simulink model "torqueControlBalancingWithSimu"  (Simulink 10.2)
settings: Solver=FixedStepDiscrete  StartTime=0.0  StopTime="Config.SIMULATION_TIME "  FixedStep=Config.tStepSim  RelTol=1e-3
PostLoadFcn:
  | %% Try to open the static GUI and try to adjust it
  | try
  | 
  |     staticGUI = simulinkStaticGUI;
  | 
  | end
InitFcn:
  | %% initialize the simulation
  | cd(fileparts(which(bdroot)));
  | initTorqueControlBalancingWithSimu;
  | 
  | %% Try to edit the GUI (the user may have already closed it)
  | try
  | 
  |     %% Update Start Button
  |     set(sl_synch_handles.startButton,'Backgroundcolor',[0.0,1.0,0.0]);
  |     set(sl_synch_handles.startButton,'Enable','on');
  | 
  | end
StartFcn:
  | %% Try to edit the GUI (the user may have already closed it)
  | try
  | 
  |     %% Update Start Button
  |     set(sl_synch_handles.startButton,'Backgroundcolor',[0.8,0.8,0.8]);
  |     set(sl_synch_handles.startButton,'Enable','off');
  | 
  |     %% Update Compile Button
  |     set(sl_synch_handles.compileButton,'Backgroundcolor',[0.8,0.8,0.8]);
  |     set(sl_synch_handles.compileButton,'Enable','off');
  | 
  |     %% Update Exit Button
  |     set(sl_synch_handles.exitButton,'Backgroundcolor',[0.8,0.8,0.8]);
  |     set(sl_synch_handles.exitButton,'Enable','off');
  | 
  | end
StopFcn:
  | %% stop the simulation
  | cd(fileparts(which(bdroot)));
  | stopTorqueControlBalancingWithSimu;
  | 
  | %% Try to edit the GUI (the user may have already closed it)
  | try
  | 
  |     %% Update Start Button
  |     if get(sl_synch_handles.checkbox_recompile, 'Value')
  |         set(sl_synch_handles.startButton,'Backgroundcolor',[0.0,1.0,0.0]);
  |         set(sl_synch_handles.startButton,'Enable','on');
  |     end
  | 
  |     %% Update Compile Button
  |     set(sl_synch_handles.compileButton,'Backgroundcolor',[1.0,0.6,0.0]);
  |     set(sl_synch_handles.compileButton,'Enable','on');
  | 
  |     %% Update Exit Button
  |     set(sl_synch_handles.exitButton,'Backgroundcolor',[0.0,1.0,1.0]);
  |     set(sl_synch_handles.exitButton,'Enable','on');
  | 
  | end
undefined symbols (not defined in the file or in its folder): bVectorConstraints, Config, confVisualizer, ConstraintsMatrix, Gain, motorsReflectedInertia, Reg, robot_config, ROBOT_DOF, Sat, StateMachine
libraries: WBToolboxLibrary x36, utilityBlocks_lib x7, mwbs_visualizers_lib x1, mwbs_robotSensors_lib x1, mwbs_robotDynamicsWithContacts_lib x1
(part 2 of 2)

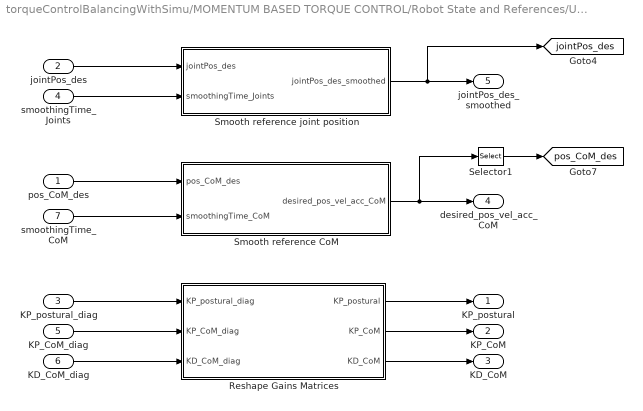
== system torqueControlBalancingWithSimu/MOMENTUM BASED TORQUE CONTROL/Robot State and References/Update Gains and References ==
  pos_CoM_des : Inport
  jointPos_des : Inport  Port=2
  KP_postural_diag : Inport  Port=3
  smoothingTime_Joints : Inport  Port=4
  KP_CoM_diag : Inport  Port=5
  KD_CoM_diag : Inport  Port=6
  smoothingTime_CoM : Inport  Port=7
  Reshape Gains Matrices : Subsystem
  Selector1 : Selector  NumberOfDimensions=2  InputPortWidth=3  IndexOptions=Index vector (dialog),Index vector (dialog)  Indices=[1 2 3],[1]  OutputSizes=1,1
  Smooth reference CoM : Subsystem
  Smooth reference joint position : Subsystem
  KP_postural : Outport  VectorParamsAs1DForOutWhenUnconnected=off
  KP_CoM : Outport  Port=2  VectorParamsAs1DForOutWhenUnconnected=off
  KD_CoM : Outport  Port=3  VectorParamsAs1DForOutWhenUnconnected=off
  desired_pos_vel_acc_CoM : Outport  Port=4  VectorParamsAs1DForOutWhenUnconnected=off
  jointPos_des_smoothed : Outport  Port=5  VectorParamsAs1DForOutWhenUnconnected=off
  tag scope: jointPos_des=global, pos_CoM_des=global
  wires:
  Smooth reference joint position/1(jointPos_des_smoothed) -> [jointPos_des], jointPos_des_smoothed/1
  jointPos_des/1 -> Smooth reference joint position/1(jointPos_des)
  smoothingTime_Joints/1 -> Smooth reference joint position/2(smoothingTime_Joints)
  pos_CoM_des/1 -> Smooth reference CoM/1(pos_CoM_des)
  smoothingTime_CoM/1 -> Smooth reference CoM/2(smoothingTime_CoM)
  Smooth reference CoM/1(desired_pos_vel_acc_CoM) -> Selector1/1, desired_pos_vel_acc_CoM/1
  KP_postural_diag/1 -> Reshape Gains Matrices/1(KP_postural_diag)
  KP_CoM_diag/1 -> Reshape Gains Matrices/2(KP_CoM_diag)
  KD_CoM_diag/1 -> Reshape Gains Matrices/3(KD_CoM_diag)
  Reshape Gains Matrices/1(KP_postural) -> KP_postural/1
  Reshape Gains Matrices/2(KP_CoM) -> KP_CoM/1
  Reshape Gains Matrices/3(KD_CoM) -> KD_CoM/1
  Selector1/1 -> [pos_CoM_des]

== system torqueControlBalancingWithSimu/MOMENTUM BASED TORQUE CONTROL/emergency stop: joint limits/STOP IF JOINTS HIT THE LIMITS ==
  jointPos : Inport
  Enable : EnablePort
  Assertion : Assertion
  GetLimits : WBToolboxLibrary/States/GetLimits  limitsSource=ControlBoard  limitsType=Position
      settings: SourceProductName=WholeBodyToolbox
  MATLAB Function : MATLAB Function  TreatAsAtomicUnit=on
  To Workspace : ToWorkspace  VariableName=res_check_range  SaveFormat=Structure With Time  SampleTime=Config.tStep
  Unit Delay : UnitDelay  InitialCondition=1  SampleTime=Config.tStep  HasFrameUpgradeWarning=on
  index1 : Constant  Value=0.01  VectorParams1D=off
  wires:
  jointPos/1 -> MATLAB Function/3(u)
  MATLAB Function/1(inRange) -> Unit Delay/1
  index1/1 -> MATLAB Function/4(tol)
  MATLAB Function/2(res_check_range) -> To Workspace/1
  Unit Delay/1 -> Assertion/1
  GetLimits/1 -> MATLAB Function/1(umin)
  GetLimits/2 -> MATLAB Function/2(umax)

== system torqueControlBalancingWithSimu/MOMENTUM BASED TORQUE CONTROL/emergency stop: joint limits/STOP IF THERE ARE SPIKES IN THE ENCODERS ==
  jointPos : Inport
  Enable : EnablePort
  Assertion : Assertion
  MATLAB Function : MATLAB Function  TreatAsAtomicUnit=on
  To Workspace : ToWorkspace  VariableName=res_check_spikes  SaveFormat=Structure With Time  SampleTime=Config.tStep
  Unit Delay : UnitDelay  InitialCondition=1  SampleTime=Config.tStep  HasFrameUpgradeWarning=on
  index1 : Constant  Value=Sat.maxJointsPositionDelta  VectorParams1D=off
  wires:
  jointPos/1 -> MATLAB Function/1(u)
  MATLAB Function/1(noSpikes) -> Unit Delay/1
  index1/1 -> MATLAB Function/2(delta_u_max)
  MATLAB Function/2(res_check_spikes) -> To Workspace/1
  Unit Delay/1 -> Assertion/1

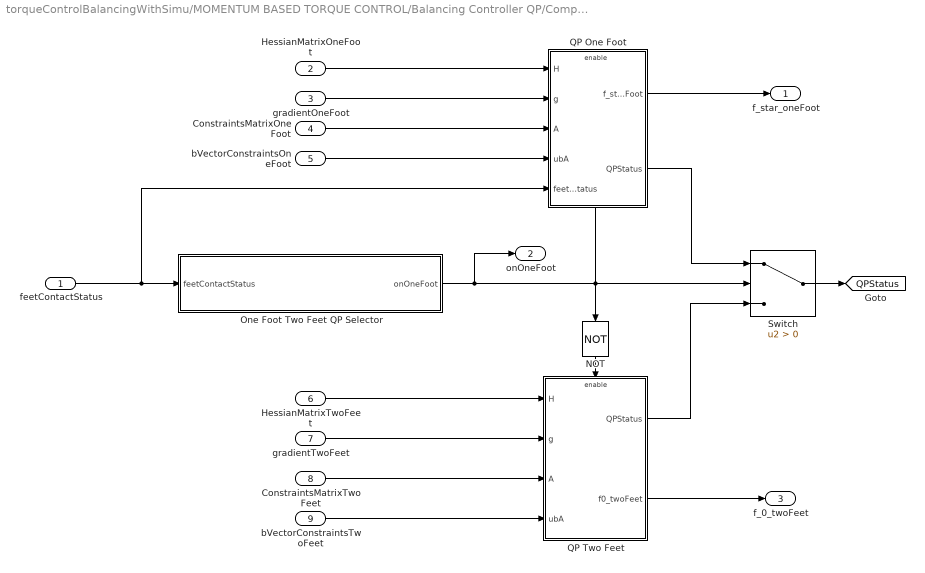
== system torqueControlBalancingWithSimu/MOMENTUM BASED TORQUE CONTROL/Balancing Controller QP/Compute Desired Torques/QPSolver ==
  feetContactStatus : Inport
  HessianMatrixOneFoot : Inport  Port=2
  gradientOneFoot : Inport  Port=3
  ConstraintsMatrixOneFoot : Inport  Port=4
  bVectorConstraintsOneFoot : Inport  Port=5
  HessianMatrixTwoFeet : Inport  Port=6
  gradientTwoFeet : Inport  Port=7
  ConstraintsMatrixTwoFeet : Inport  Port=8
  bVectorConstraintsTwoFeet : Inport  Port=9
  NOT : Logic  Operator=NOT  IconShape=distinctive  AllPortsSameDT=off  OutDataTypeStr=boolean
  One Foot Two Feet QP Selector : MATLAB Function  TreatAsAtomicUnit=on
  QP One Foot : Subsystem  TreatAsAtomicUnit=on
  QP Two Feet : Subsystem  TreatAsAtomicUnit=on
  Switch : Switch  Criteria=u2 > Threshold
  f_star_oneFoot : Outport  VectorParamsAs1DForOutWhenUnconnected=off
  onOneFoot : Outport  Port=2  VectorParamsAs1DForOutWhenUnconnected=off
  f_0_twoFeet : Outport  Port=3  VectorParamsAs1DForOutWhenUnconnected=off
  tag scope: QPStatus=global
  wires:
  feetContactStatus/1 -> QP One Foot/5(feetContactStatus), One Foot Two Feet QP Selector/1(feetContactStatus)
  HessianMatrixOneFoot/1 -> QP One Foot/1(H)
  bVectorConstraintsTwoFeet/1 -> QP Two Feet/4(ubA)
  gradientOneFoot/1 -> QP One Foot/2(g)
  ConstraintsMatrixOneFoot/1 -> QP One Foot/3(A)
  gradientTwoFeet/1 -> QP Two Feet/2(g)
  ConstraintsMatrixTwoFeet/1 -> QP Two Feet/3(A)
  bVectorConstraintsOneFoot/1 -> QP One Foot/4(ubA)
  HessianMatrixTwoFeet/1 -> QP Two Feet/1(H)
  QP One Foot/2(QPStatus) -> Switch/1
  QP Two Feet/1(QPStatus) -> Switch/3
  QP Two Feet/2(f0_twoFeet) -> f_0_twoFeet/1
  NOT/1 -> QP Two Feet/Enable
  One Foot Two Feet QP Selector/1(onOneFoot) -> onOneFoot/1, NOT/1, Switch/2, QP One Foot/Enable
  QP One Foot/1(f_star_oneFoot) -> f_star_oneFoot/1
  Switch/1 -> [QPStatus]

== system torqueControlBalancingWithSimu/MOMENTUM BASED TORQUE CONTROL/Balancing Controller QP/Compute angular momentum integral error/Compute base to fixed link transform ==
  jointPos : Inport
  Constant7 : Constant  Value=eye(4)
  "inv  " : Product  Inputs=/  Multiplication=Matrix(*)
  inv  1 : Product  Inputs=/  Multiplication=Matrix(*)
  l_sole to root_link relative transform : WBToolboxLibrary/Model/Kinematics/ForwardKinematics  frameName=Frames.LEFT_FOOT
      settings: SourceProductName=WholeBodyToolbox
  r_sole to root_link relative transform : WBToolboxLibrary/Model/Kinematics/ForwardKinematics  frameName=Frames.RIGHT_FOOT
      settings: SourceProductName=WholeBodyToolbox
  fixed_l_sole_H_b : Outport  VectorParamsAs1DForOutWhenUnconnected=off
  fixed_r_sole_H_b : Outport  Port=2  VectorParamsAs1DForOutWhenUnconnected=off
  wires:
  Constant7/1 -> l_sole to root_link relative transform/1, r_sole to root_link relative transform/1
  inv  1/1 -> fixed_r_sole_H_b/1
  "inv  "/1 -> fixed_l_sole_H_b/1
  jointPos/1 -> r_sole to root_link relative transform/2, l_sole to root_link relative transform/2
  l_sole to root_link relative transform/1 -> "inv  "/1
  r_sole to root_link relative transform/1 -> inv  1/1

== system torqueControlBalancingWithSimu/MOMENTUM BASED TORQUE CONTROL/Dump and visualize/Desired and Measured Forces/Demux Forces nd Moments ==
  wrench_leftFoot : Inport
  wrench_rightFoot : Inport  Port=2
  f_star : Inport  Port=3
  Demux{1,5..7} (4 alike) : Demux  Outputs=[3;3]
  Demux2 : Demux  Outputs=[6;6]
  measured forces l_sole : Outport  VectorParamsAs1DForOutWhenUnconnected=off
  des forces l_sole : Outport  Port=2  VectorParamsAs1DForOutWhenUnconnected=off
  measured forces r_sole : Outport  Port=3  VectorParamsAs1DForOutWhenUnconnected=off
  des forces r_sole : Outport  Port=4  VectorParamsAs1DForOutWhenUnconnected=off
  measured moments l_sole : Outport  Port=5  VectorParamsAs1DForOutWhenUnconnected=off
  des moments l_sole : Outport  Port=6  VectorParamsAs1DForOutWhenUnconnected=off
  measured moments r_sole : Outport  Port=7  VectorParamsAs1DForOutWhenUnconnected=off
  des moments r_sole : Outport  Port=8  VectorParamsAs1DForOutWhenUnconnected=off
  wires:
  Demux6/2 -> des moments r_sole/1
  Demux5/2 -> des moments l_sole/1
  Demux1/1 -> measured forces l_sole/1
  Demux7/1 -> measured forces r_sole/1
  Demux7/2 -> measured moments r_sole/1
  wrench_leftFoot/1 -> Demux1/1
  Demux2/1 -> Demux5/1
  wrench_rightFoot/1 -> Demux7/1
  Demux6/1 -> des forces r_sole/1
  Demux1/2 -> measured moments l_sole/1
  f_star/1 -> Demux2/1
  Demux2/2 -> Demux6/1
  Demux5/1 -> des forces l_sole/1

== system torqueControlBalancingWithSimu/MOMENTUM BASED TORQUE CONTROL/Dynamics and Kinematics/Dynamics/Add motors reflected inertia ==
  M : Inport
  Add motor reflected inertias : MATLAB Function  TreatAsAtomicUnit=on
  Constant : Constant  Value=Config.USE_MOTOR_REFLECTED_INERTIA
  Switch : Switch  Criteria=u2 > Threshold
  M_with_motor_inertia : Outport  VectorParamsAs1DForOutWhenUnconnected=off
  wires:
  M/1 -> Switch/3, Add motor reflected inertias/1(M)
  Constant/1 -> Switch/2
  Add motor reflected inertias/1(M_with_inertia) -> Switch/1
  Switch/1 -> M_with_motor_inertia/1

== system torqueControlBalancingWithSimu/MOMENTUM BASED TORQUE CONTROL/Robot State and References/Compute State Velocity/Feet Jacobians ==
  jointPos : Inport
  w_H_b : Inport  Port=2
  Jacobian l_sole : WBToolboxLibrary/Model/Jacobians/Jacobian  frameName=Frames.LEFT_FOOT
      settings: SourceProductName=WholeBodyToolbox
  Jacobian r_sole : WBToolboxLibrary/Model/Jacobians/Jacobian  frameName=Frames.RIGHT_FOOT
      settings: SourceProductName=WholeBodyToolbox
  J_l_sole : Outport  VectorParamsAs1DForOutWhenUnconnected=off
  J_r_sole : Outport  Port=2  VectorParamsAs1DForOutWhenUnconnected=off
  wires:
  Jacobian l_sole/1 -> J_l_sole/1
  Jacobian r_sole/1 -> J_r_sole/1
  w_H_b/1 -> Jacobian r_sole/1, Jacobian l_sole/1
  jointPos/1 -> Jacobian l_sole/2, Jacobian r_sole/2

== system torqueControlBalancingWithSimu/MOMENTUM BASED TORQUE CONTROL/Robot State and References/Compute base to fixed link transform/LFoot to base link transform  ==
  neck_pos : Inport
  jointPos : Inport  Port=2
  inertial : Inport  Port=3
  w_H_link : Inport  Port=4
  w_H_base_fixed : Inport  Port=5
  Fixe d base to root link transform : WBToolboxLibrary/Model/Kinematics/ForwardKinematics  frameName=Frames.BASE
      settings: SourceProductName=WholeBodyToolbox
  Fixed base to imu transform : WBToolboxLibrary/Model/Kinematics/ForwardKinematics  frameName=Frames.IMU
      settings: SourceProductName=WholeBodyToolbox
  Get Base Rotation From IMU : MATLAB Function  TreatAsAtomicUnit=on
  Inv : Product  Inputs=/*  Multiplication=Matrix(*)
  Inv_2 : Product  Inputs=/*  Multiplication=Matrix(*)
  Selector1 : Selector  InputPortWidth=Ports.IMU_PORT_SIZE  IndexOptions=Index vector (dialog)  Indices=Ports.IMU_PORT_ORIENTATION_INDEX  OutputSizes=1
  Selector2 : Selector  InputPortWidth=Ports.IMU_PORT_SIZE  IndexOptions=Index vector (dialog)  Indices=Ports.IMU_PORT_ORIENTATION_INDEX  OutputSizes=1
  Switch6 : Switch  Criteria=u2 > Threshold
  USE_IMU4EST_BASE : Constant  Value=Config.USE_IMU4EST_BASE
  holder 1 : utilityBlocks_lib/Holder  SystemSampleTime=Config.tStep  VariantActivationTime=update diagram  Latency=0  AutoFrameSizeCalculation=off
      settings: SourceProductName=WholeBodyControllers
  holder 2 : utilityBlocks_lib/Holder  SystemSampleTime=Config.tStep  VariantActivationTime=update diagram  Latency=0  AutoFrameSizeCalculation=off
      settings: SourceProductName=WholeBodyControllers
  neck transform : Subsystem
  link_H_b : Outport  VectorParamsAs1DForOutWhenUnconnected=off
  wires:
  Switch6/1 -> link_H_b/1
  Inv_2/1 -> Switch6/3, Get Base Rotation From IMU/3(fixedLink_H_base)  "link_H_root"
  USE_IMU4EST_BASE/1 -> Switch6/2
  Inv/1 -> holder 1/1, Get Base Rotation From IMU/1(imu_H_fixedLink)  "imu_H_link"
  holder 2/1 -> Selector2/1
  Fixed base to imu transform/1 -> Inv/1
  jointPos/1 -> Fixed base to imu transform/2, Fixe d base to root link transform/2
  Get Base Rotation From IMU/1(w_H_b) -> Switch6/1
  Fixe d base to root link transform/1 -> Inv_2/2
  inertial/1 -> Selector1/1, holder 2/1
  neck_pos/1 -> neck transform/1(neck port)
  w_H_link/1 -> Inv_2/1, Inv/2
  w_H_base_fixed/1 -> Fixe d base to root link transform/1, Fixed base to imu transform/1
  Selector2/1 -> Get Base Rotation From IMU/4(rpyFromIMU_0)
  holder 1/1 -> Get Base Rotation From IMU/2(imu_H_fixedLink_0)
  Selector1/1 -> Get Base Rotation From IMU/5(rpyFromIMU)
  neck transform/1(neck position) -> Get Base Rotation From IMU/6(neck_pos)

== system torqueControlBalancingWithSimu/MOMENTUM BASED TORQUE CONTROL/Robot State and References/Compute base to fixed link transform/RFoot to base link transform ==
  neck_pos : Inport
  jointPos : Inport  Port=2
  inertial : Inport  Port=3
  w_H_link : Inport  Port=4
  w_H_base_fixed : Inport  Port=5
  Fixed base to imu transform : WBToolboxLibrary/Model/Kinematics/ForwardKinematics  frameName=Frames.IMU
      settings: SourceProductName=WholeBodyToolbox
  Fixed base to root link transform : WBToolboxLibrary/Model/Kinematics/ForwardKinematics  frameName=Frames.BASE
      settings: SourceProductName=WholeBodyToolbox
  Get Base Rotation From IMU : MATLAB Function  TreatAsAtomicUnit=on
  Inv : Product  Inputs=/*  Multiplication=Matrix(*)
  Inv_2 : Product  Inputs=/*  Multiplication=Matrix(*)
  Selector1 : Selector  InputPortWidth=Ports.IMU_PORT_SIZE  IndexOptions=Index vector (dialog)  Indices=Ports.IMU_PORT_ORIENTATION_INDEX  OutputSizes=1
  Selector2 : Selector  InputPortWidth=Ports.IMU_PORT_SIZE  IndexOptions=Index vector (dialog)  Indices=Ports.IMU_PORT_ORIENTATION_INDEX  OutputSizes=1
  Switch6 : Switch  Criteria=u2 > Threshold
  USE_IMU4EST_BASE : Constant  Value=Config.USE_IMU4EST_BASE
  holder 3 : utilityBlocks_lib/Holder  SystemSampleTime=Config.tStep  VariantActivationTime=update diagram  Latency=0  AutoFrameSizeCalculation=off
      settings: SourceProductName=WholeBodyControllers
  holder 4 : utilityBlocks_lib/Holder  SystemSampleTime=Config.tStep  VariantActivationTime=update diagram  Latency=0  AutoFrameSizeCalculation=off
      settings: SourceProductName=WholeBodyControllers
  neck transform : Subsystem
  link_H_b : Outport  VectorParamsAs1DForOutWhenUnconnected=off
  wires:
  Switch6/1 -> link_H_b/1
  Inv_2/1 -> Switch6/3, Get Base Rotation From IMU/3(fixedLink_H_base)  "link_H_root"
  USE_IMU4EST_BASE/1 -> Switch6/2
  Inv/1 -> holder 3/1, Get Base Rotation From IMU/1(imu_H_fixedLink)  "imu_H_link"
  holder 4/1 -> Selector2/1
  Fixed base to imu transform/1 -> Inv/1
  jointPos/1 -> Fixed base to imu transform/2, Fixed base to root link transform/2
  Get Base Rotation From IMU/1(w_H_b) -> Switch6/1
  Fixed base to root link transform/1 -> Inv_2/2
  inertial/1 -> holder 4/1, Selector1/1
  neck_pos/1 -> neck transform/1(neck port)
  neck transform/1(neck position) -> Get Base Rotation From IMU/6(neck_pos)
  w_H_link/1 -> Inv_2/1, Inv/2
  w_H_base_fixed/1 -> Fixed base to root link transform/1, Fixed base to imu transform/1
  Selector2/1 -> Get Base Rotation From IMU/4(rpyFromIMU_0)
  holder 3/1 -> Get Base Rotation From IMU/2(imu_H_fixedLink_0)
  Selector1/1 -> Get Base Rotation From IMU/5(rpyFromIMU)

== system torqueControlBalancingWithSimu/MOMENTUM BASED TORQUE CONTROL/Robot State and References/State Machine/xCom ==
  w_H_b : Inport
  jointPos : Inport  Port=2
  CoM : WBToolboxLibrary/Model/Kinematics/ForwardKinematics  frameName=Frames.COM
      settings: SourceProductName=WholeBodyToolbox
  "CoM6D ->  CoMXYZ2" : Selector  NumberOfDimensions=2  InputPortWidth=7  IndexOptions=Index vector (dialog),Index vector (dialog)  Indices=[1 2 3],[4]  OutputSizes=1,1
  "pos_CoM_fixed_l_sole " : Outport  VectorParamsAs1DForOutWhenUnconnected=off
  wires:
  jointPos/1 -> CoM/2
  "CoM6D ->  CoMXYZ2"/1 -> "pos_CoM_fixed_l_sole "/1
  CoM/1 -> "CoM6D ->  CoMXYZ2"/1
  w_H_b/1 -> CoM/1

== system torqueControlBalancingWithSimu/MOMENTUM BASED TORQUE CONTROL/Robot State and References/State Machine/xCom2 ==
  w_H_b : Inport
  jointPos : Inport  Port=2
  CoM : WBToolboxLibrary/Model/Kinematics/ForwardKinematics  frameName=Frames.COM
      settings: SourceProductName=WholeBodyToolbox
  "CoM6D ->  CoMXYZ2" : Selector  NumberOfDimensions=2  InputPortWidth=7  IndexOptions=Index vector (dialog),Index vector (dialog)  Indices=[1 2 3],[4]  OutputSizes=1,1
  "pos_CoM_fixed_r_sole " : Outport  VectorParamsAs1DForOutWhenUnconnected=off
  wires:
  jointPos/1 -> CoM/2
  "CoM6D ->  CoMXYZ2"/1 -> "pos_CoM_fixed_r_sole "/1
  CoM/1 -> "CoM6D ->  CoMXYZ2"/1
  w_H_b/1 -> CoM/1

== system torqueControlBalancingWithSimu/MOMENTUM BASED TORQUE CONTROL/Robot State and References/Update Gains and References/Reshape Gains Matrices ==
  KP_postural_diag : Inport
  KP_CoM_diag : Inport  Port=2
  KD_CoM_diag : Inport  Port=3
  MATLAB Function : MATLAB Function  TreatAsAtomicUnit=on
  MATLAB Function1 : MATLAB Function  TreatAsAtomicUnit=on
  MATLAB Function2 : MATLAB Function  TreatAsAtomicUnit=on
  KP_postural : Outport  VectorParamsAs1DForOutWhenUnconnected=off
  KP_CoM : Outport  Port=2  VectorParamsAs1DForOutWhenUnconnected=off
  KD_CoM : Outport  Port=3  VectorParamsAs1DForOutWhenUnconnected=off
  wires:
  KP_postural_diag/1 -> MATLAB Function/1(d)
  KP_CoM_diag/1 -> MATLAB Function1/1(d)
  KD_CoM_diag/1 -> MATLAB Function2/1(d)
  MATLAB Function/1(D) -> KP_postural/1
  MATLAB Function1/1(D) -> KP_CoM/1
  MATLAB Function2/1(D) -> KD_CoM/1

== system torqueControlBalancingWithSimu/MOMENTUM BASED TORQUE CONTROL/Robot State and References/Update Gains and References/Smooth reference CoM ==
  pos_CoM_des : Inport
  smoothingTime_CoM : Inport  Port=2
  Constant : Constant  Value=zeros(6,1)
  MinimumJerkTrajectoryGenerator2 : WBToolboxLibrary/Utilities/MinimumJerkTrajectoryGenerator  externalSettlingTime=on  settlingTime=0.01  sampleTime=Config.tStep  resetOnSettlingTime=off  firstDerivatives=on  secondDerivatives=on  explicitInitialValue=off
      settings: SourceProductName=WholeBodyToolbox
  Mux : Mux  Inputs=3
  Mux1 : Mux  Inputs=2
  Reshape : Reshape  OutputDimensionality=Customize  OutputDimensions=[3,3]
  SMOOTH_DES_COM : Constant  Value=Config.SMOOTH_COM_DES
  Switch3 : Switch  Criteria=u2 > Threshold
  desired_pos_vel_acc_CoM : Outport  VectorParamsAs1DForOutWhenUnconnected=off
  wires:
  smoothingTime_CoM/1 -> MinimumJerkTrajectoryGenerator2/2
  Switch3/1 -> Reshape/1
  pos_CoM_des/1 -> Mux1/1, MinimumJerkTrajectoryGenerator2/1
  SMOOTH_DES_COM/1 -> Switch3/2
  MinimumJerkTrajectoryGenerator2/3 -> Mux/3
  Mux/1 -> Switch3/1
  MinimumJerkTrajectoryGenerator2/2 -> Mux/2
  Reshape/1 -> desired_pos_vel_acc_CoM/1
  MinimumJerkTrajectoryGenerator2/1 -> Mux/1
  Mux1/1 -> Switch3/3
  Constant/1 -> Mux1/2

== system torqueControlBalancingWithSimu/MOMENTUM BASED TORQUE CONTROL/Robot State and References/Update Gains and References/Smooth reference joint position ==
  jointPos_des : Inport
  smoothingTime_Joints : Inport  Port=2
  MinimumJerkTrajectoryGenerator1 : WBToolboxLibrary/Utilities/MinimumJerkTrajectoryGenerator  externalSettlingTime=on  settlingTime=0.01  sampleTime=Config.tStep  resetOnSettlingTime=off  firstDerivatives=on  secondDerivatives=on  explicitInitialValue=off
      settings: SourceProductName=WholeBodyToolbox
  SMOOTH_DES_COM2 : Constant  Value=Config.SMOOTH_JOINT_DES
  Switch5 : Switch  Criteria=u2 > Threshold
  Terminator : Terminator
  jointPos_des_smoothed : Outport  VectorParamsAs1DForOutWhenUnconnected=off
  tag scope: jointAcc_des=global
  wires:
  SMOOTH_DES_COM2/1 -> Switch5/2
  Switch5/1 -> jointPos_des_smoothed/1
  jointPos_des/1 -> MinimumJerkTrajectoryGenerator1/1, Switch5/3
  smoothingTime_Joints/1 -> MinimumJerkTrajectoryGenerator1/2
  MinimumJerkTrajectoryGenerator1/1 -> Switch5/1
  MinimumJerkTrajectoryGenerator1/3 -> [jointAcc_des]
  MinimumJerkTrajectoryGenerator1/2 -> Terminator/1

== system torqueControlBalancingWithSimu/MOMENTUM BASED TORQUE CONTROL/Balancing Controller QP/Compute Desired Torques/QPSolver/QP One Foot ==
  H : Inport
  g : Inport  Port=2
  A : Inport  Port=3
  ubA : Inport  Port=4
  feetContactStatus : Inport  Port=5
  Enable : EnablePort
  Analytical Solution QP One Foot (unconstrained) : MATLAB Function  TreatAsAtomicUnit=on
  Constant : Constant  Value=-Inf(19,1)
  MatchSignalSizes : WBToolboxLibrary/Utilities/MatchSignalSizes
      settings: SourceProductName=WholeBodyToolbox
  Process QP output : MATLAB Function  TreatAsAtomicUnit=on
  QP One Foot : WBToolboxLibrary/Utilities/QP  lbA=on  ubA=on  lb=off  ub=off  computeObjVal=off  stopIfFails=off
      settings: SourceProductName=WholeBodyToolbox
  f_star_oneFoot : Outport  VectorParamsAs1DForOutWhenUnconnected=off
  QPStatus : Outport  Port=2  VectorParamsAs1DForOutWhenUnconnected=off
  wires:
  MatchSignalSizes/1 -> Process QP output/2(primalSolution)
  A/1 -> QP One Foot/3
  H/1 -> Analytical Solution QP One Foot (unconstrained)/1(H), QP One Foot/1
  ubA/1 -> QP One Foot/5
  g/1 -> Analytical Solution QP One Foot (unconstrained)/2(g), MatchSignalSizes/1, QP One Foot/2
  Analytical Solution QP One Foot (unconstrained)/1(analyticalSolution) -> Process QP output/1(analyticalSolution)
  QP One Foot/2 -> Process QP output/3(QPStatus), QPStatus/1
  QP One Foot/1 -> MatchSignalSizes/2
  feetContactStatus/1 -> Process QP output/4(feetContactStatus)
  Process QP output/1(f_star) -> f_star_oneFoot/1
  Constant/1 -> QP One Foot/4

== system torqueControlBalancingWithSimu/MOMENTUM BASED TORQUE CONTROL/Balancing Controller QP/Compute Desired Torques/QPSolver/QP Two Feet ==
  H : Inport
  g : Inport  Port=2
  A : Inport  Port=3
  ubA : Inport  Port=4
  Enable : EnablePort
  Analytical Solution Two Feet (unconstrained) : MATLAB Function  TreatAsAtomicUnit=on
  Constant : Constant  Value=-Inf(38,1)
  MatchSignalSizes : WBToolboxLibrary/Utilities/MatchSignalSizes
      settings: SourceProductName=WholeBodyToolbox
  Process QP output : MATLAB Function  TreatAsAtomicUnit=on
  QP Two Feet : WBToolboxLibrary/Utilities/QP  lbA=on  ubA=on  lb=off  ub=off  computeObjVal=off  stopIfFails=off
      settings: SourceProductName=WholeBodyToolbox
  QPStatus : Outport  VectorParamsAs1DForOutWhenUnconnected=off
  f0_twoFeet : Outport  Port=2  VectorParamsAs1DForOutWhenUnconnected=off
  wires:
  QP Two Feet/2 -> QPStatus/1, Process QP output/3(QPStatus)
  A/1 -> QP Two Feet/3
  Analytical Solution Two Feet (unconstrained)/1(analyticalSolution) -> Process QP output/1(analyticalSolution)
  Process QP output/1(f_star) -> f0_twoFeet/1
  MatchSignalSizes/1 -> Process QP output/2(primalSolution)
  QP Two Feet/1 -> MatchSignalSizes/2
  H/1 -> Analytical Solution Two Feet (unconstrained)/1(H), QP Two Feet/1
  g/1 -> Analytical Solution Two Feet (unconstrained)/2(g), MatchSignalSizes/1, QP Two Feet/2
  ubA/1 -> QP Two Feet/5
  Constant/1 -> QP Two Feet/4

== system torqueControlBalancingWithSimu/MOMENTUM BASED TORQUE CONTROL/Robot State and References/Compute base to fixed link transform/LFoot to base link transform /neck transform ==
  neck port : Inport
  Constant : Constant  Value=zeros(3,1)
  Switch : Switch  Criteria=u2 > Threshold
  USE_IMU4EST_BASE1 : Constant  Value=Config.CORRECT_NECK_IMU
  neck position : Outport  VectorParamsAs1DForOutWhenUnconnected=off
  wires:
  USE_IMU4EST_BASE1/1 -> Switch/2
  Switch/1 -> neck position/1
  Constant/1 -> Switch/3
  neck port/1 -> Switch/1  "neck pos"

== system torqueControlBalancingWithSimu/MOMENTUM BASED TORQUE CONTROL/Robot State and References/Compute base to fixed link transform/RFoot to base link transform/neck transform ==
  neck port : Inport
  Constant : Constant  Value=zeros(3,1)
  Switch : Switch  Criteria=u2 > Threshold
  USE_IMU4EST_BASE1 : Constant  Value=Config.CORRECT_NECK_IMU
  neck position : Outport  VectorParamsAs1DForOutWhenUnconnected=off
  wires:
  USE_IMU4EST_BASE1/1 -> Switch/2
  Switch/1 -> neck position/1
  Constant/1 -> Switch/3
  neck port/1 -> Switch/1  "neck pos"

== matlab function MOMENTUM BASED TORQUE CONTROL/Robot State and References/Update Gains and References/Reshape Gains Matrices/MATLAB Function1 ==
  data: d input double; D output double
function D = diagonalMatrixFromVectorFCN(d)

    D = wbc.diagonalMatrixFromVector(d);
end

== matlab function MOMENTUM BASED TORQUE CONTROL/Robot State and References/Update Gains and References/Reshape Gains Matrices/MATLAB Function ==
  data: d input double; D output double
function D = diagonalMatrixFromVectorFCN(d)

    D = wbc.diagonalMatrixFromVector(d);
end

== matlab function MOMENTUM BASED TORQUE CONTROL/Robot State and References/Compute base to fixed link transform/RFoot to base link transform/Get Base Rotation From IMU ==
  data: imu_H_fixedLink input double; imu_H_fixedLink_0 input double; fixedLink_H_base input double; rpyFromIMU_0 input double; rpyFromIMU input double; neck_pos input double; w_H_b output double; Config parameter double
function w_H_b = getWorldToBaseTransformFCN(imu_H_fixedLink, imu_H_fixedLink_0, fixedLink_H_base, rpyFromIMU_0, rpyFromIMU, neck_pos, Config)

    FILTER_IMU_YAW = Config.FILTER_IMU_YAW;
    
    [w_H_b, wImu_H_base, wImu_H_fixedLink_0] = wbc.worldToBaseTransformWithIMU(imu_H_fixedLink, imu_H_fixedLink_0, fixedLink_H_base, rpyFromIMU_0, rpyFromIMU, FILTER_IMU_YAW);
    
    % Correct head IMU with neck positions (HEAD IMU only)
    if Config.CORRECT_NECK_IMU
        
        wImu_H_wImuAssumingNeckToZero = wbc.correctIMUWithNeckPos(neck_pos);
        wImu_H_base                   = wImu_H_wImuAssumingNeckToZero * wImu_H_base;
        w_H_b                         = wImu_H_fixedLink_0\wImu_H_base;  
    end
end

== matlab function MOMENTUM BASED TORQUE CONTROL/Robot State and References/Update Gains and References/Reshape Gains Matrices/MATLAB Function2 ==
  data: d input double; D output double
function D = diagonalMatrixFromVectorFCN(d)

    D = wbc.diagonalMatrixFromVector(d);
end

== matlab function Subsystem/MATLAB Function ==
  data: jointVelocities input double; motorJointTorques input double; jointTorques output double; jointFrictionMat parameter double
function jointTorques = frictionModel(jointVelocities,motorJointTorques,jointFrictionMat)

jointTorques = motorJointTorques - jointFrictionMat*jointVelocities;

== matlab function MOMENTUM BASED TORQUE CONTROL/Dynamics and Kinematics/Dynamics/Add motors reflected inertia/Add motor reflected inertias ==
  data: M input double; M_with_inertia output double; Config parameter double
function M_with_inertia = addMotorsInertiaFCN(M,Config)

    Gamma = Config.Gamma;
    T     = Config.T;
    I_m   = Config.I_m;
    
    M_with_inertia = wbc.addMotorsReflectedInertia(M,Gamma,T,I_m);
end

== matlab function MOMENTUM BASED TORQUE CONTROL/Robot State and References/Compute State Velocity/Compute Base Velocity ==
  data: J_l_sole input double; J_r_sole input double; feetContactStatus input double; nu_b output double; jointVel input double; Reg parameter double
function nu_b = computeBaseVelocityFCN(J_l_sole, J_r_sole, feetContactStatus, jointVel, Reg)

    pinvDamp_baseVel = Reg.pinvDamp_baseVel;
    
    nu_b = wbc.computeBaseVelocityWithFeetContact(J_l_sole, J_r_sole, feetContactStatus, jointVel, pinvDamp_baseVel);
end

== matlab function MOMENTUM BASED TORQUE CONTROL/Robot State and References/Compute base to fixed link transform/LFoot to base link transform /Get Base Rotation From IMU ==
  data: imu_H_fixedLink input double; imu_H_fixedLink_0 input double; fixedLink_H_base input double; rpyFromIMU_0 input double; rpyFromIMU input double; neck_pos input double; w_H_b output double; Config parameter double
function w_H_b = getWorldToBaseTransformFCN(imu_H_fixedLink, imu_H_fixedLink_0, fixedLink_H_base, rpyFromIMU_0, rpyFromIMU, neck_pos, Config)

    FILTER_IMU_YAW = Config.FILTER_IMU_YAW;
    
    [w_H_b, wImu_H_base, wImu_H_fixedLink_0] = wbc.worldToBaseTransformWithIMU(imu_H_fixedLink, imu_H_fixedLink_0, fixedLink_H_base, rpyFromIMU_0, rpyFromIMU, FILTER_IMU_YAW);
    
    % Correct head IMU with neck positions (HEAD IMU only)
    if Config.CORRECT_NECK_IMU
        
        wImu_H_wImuAssumingNeckToZero = wbc.correctIMUWithNeckPos(neck_pos);
        wImu_H_base                   = wImu_H_wImuAssumingNeckToZero * wImu_H_base;
        w_H_b                         = wImu_H_fixedLink_0\wImu_H_base;  
    end
end

== matlab function MOMENTUM BASED TORQUE CONTROL/Balancing Controller QP/From tau_QP to Joint Torques (motor reflected inertia)/(transpose(T*Gamma))^{-1}*I_m*(T*Gamma)^{-1} ==
  data: reflectedInertia output double; Config parameter double
function reflectedInertia  = computeMotorsInertiaFCN(Config)
    
    Gamma = Config.Gamma;
    T     = Config.T;
    I_m   = Config.I_m;
    
    reflectedInertia = wbc.computeMotorsReflectedInertia(Gamma,T,I_m);
end

== matlab function MOMENTUM BASED TORQUE CONTROL/MATLAB Function ==
  data: M input double; conditionNumber output double
function conditionNumber = matConditionNumber(M)

conditionNumber = cond(M);

== matlab function MOMENTUM BASED TORQUE CONTROL/Joint Torque Saturation/Saturate Torque Derivative ==
  data: u input double; uSat output double; u_0 input double; tStep input double; uDotMax input double
function uSat = saturateInputDerivativeFCN(u, u_0, tStep, uDotMax)

    uSat = wbc.saturateInputDerivative(u, u_0, tStep, uDotMax);
end

== matlab function MOMENTUM BASED TORQUE CONTROL/Robot State and References/State Machine/STATE MACHINE ==
  data: pos_CoM_0 input double; jointPos_0 input double; pos_CoM_fixed_l_sole input double; pos_CoM_fixed_r_sole input double; jointPos input double; time input double; wrench_rightFoot input double; wrench_leftFoot input double; w_H_b output double; pos_CoM_des output double; jointPos_des output double; feetContactStatus output double; l_sole_H_b input double; r_sole_H_b input double; StateMachine parameter double; KP_postural_diag output double; KP_CoM_diag output double; KD_CoM_diag output double; Gain parameter double; state output double; smoothingTimeJoints output double; smoothingTimeCoM output double; Config parameter double
function [w_H_b, pos_CoM_des, jointPos_des, feetContactStatus, KP_postural_diag, KP_CoM_diag, KD_CoM_diag, state, smoothingTimeJoints, smoothingTimeCoM] = ...
              stateMachineMomentumControlFCN(pos_CoM_0, jointPos_0, pos_CoM_fixed_l_sole, pos_CoM_fixed_r_sole, jointPos, ...
                                             time, wrench_rightFoot, wrench_leftFoot, l_sole_H_b, r_sole_H_b, StateMachine, Gain, Config)
 
    [w_H_b, pos_CoM_des, jointPos_des, feetContactStatus, KP_postural_diag, KP_CoM_diag, KD_CoM_diag, state, smoothingTimeJoints, smoothingTimeCoM] = ...
        stateMachineMomentumControl(pos_CoM_0, jointPos_0, pos_CoM_fixed_l_sole, pos_CoM_fixed_r_sole, jointPos, ...
                                    time, wrench_rightFoot, wrench_leftFoot, l_sole_H_b, r_sole_H_b, StateMachine, Gain, Config);
end

== matlab function MOMENTUM BASED TORQUE CONTROL/emergency stop: joint limits/STOP IF THERE ARE SPIKES IN THE ENCODERS/MATLAB Function ==
  data: u input double; delta_u_max input double; noSpikes output double; res_check_spikes output double
function [noSpikes, res_check_spikes] = checkInputSpikesFCN(u, delta_u_max)

     [noSpikes, res_check_spikes] = wbc.checkInputSpikes(u, delta_u_max);
end

== matlab function MOMENTUM BASED TORQUE CONTROL/Balancing Controller QP/Compute Desired Torques/QPSolver/One Foot Two Feet QP Selector ==
  data: feetContactStatus input double; onOneFoot output double
function onOneFoot = robotIsOnSingleSupportQP_FCN(feetContactStatus)

    onOneFoot = wbc.robotIsOnSingleSupportQP(feetContactStatus);
end

== matlab function MOMENTUM BASED TORQUE CONTROL/Balancing Controller QP/Momentum Based Balancing Controller  ==
  data: HessianMatrixOneFoot output double; gradientOneFoot output double; ConstraintsMatrixOneFoot output double; bVectorConstraintsOneFoot output double; HessianMatrixTwoFeet output double; gradientTwoFeet output double; ConstraintsMatrixTwoFeet output double; bVectorConstraintsTwoFeet output double; tauModel output double; Sigma output double; Na output double; f_LDot output double; feetContactStatus input double; ConstraintsMatrix input double; bVectorConstraints input double; jointPos input double; jointPos_des input double; nu input double; M input double; h input double; L input double; intL_angMomError input double; w_H_l_sole input double; w_H_r_sole input double; J_l_sole input double; J_r_sole input double; JDot_l_sole_nu input double; JDot_r_sole_nu input double; pos_CoM input double; J_CoM input double; desired_pos_vel_acc_CoM input double; KP_CoM input double; KD_CoM input double; KP_postural input double; Reg parameter double; Gain parameter double; Config parameter double
function [HessianMatrixOneFoot, gradientOneFoot, ConstraintsMatrixOneFoot, bVectorConstraintsOneFoot, ...
          HessianMatrixTwoFeet, gradientTwoFeet, ConstraintsMatrixTwoFeet, bVectorConstraintsTwoFeet, ...
          tauModel, Sigma, Na, f_LDot] =  ...
              momentumBasedControllerFCN(feetContactStatus, ConstraintsMatrix, bVectorConstraints, jointPos, jointPos_des, nu, M, h, L, intL_angMomError, w_H_l_sole, w_H_r_sole, ...
                                         J_l_sole, J_r_sole, JDot_l_sole_nu, JDot_r_sole_nu, pos_CoM, J_CoM, desired_pos_vel_acc_CoM, KP_CoM, KD_CoM, KP_postural, Reg, Gain, Config)
                                                 
    [HessianMatrixOneFoot, gradientOneFoot, ConstraintsMatrixOneFoot, bVectorConstraintsOneFoot, ...
     HessianMatrixTwoFeet, gradientTwoFeet, ConstraintsMatrixTwoFeet, bVectorConstraintsTwoFeet, ...
     tauModel, Sigma, Na, f_LDot] =  ...
        momentumBasedController(feetContactStatus, ConstraintsMatrix, bVectorConstraints, jointPos, jointPos_des, nu, M, h, L, intL_angMomError, w_H_l_sole, w_H_r_sole, ...
                                J_l_sole, J_r_sole, JDot_l_sole_nu, JDot_r_sole_nu, pos_CoM, J_CoM, desired_pos_vel_acc_CoM, KP_CoM, KD_CoM, KP_postural, Config, Reg, Gain);
end

== matlab function MOMENTUM BASED TORQUE CONTROL/emergency stop: joint limits/STOP IF JOINTS HIT THE LIMITS/MATLAB Function ==
  data: umin input double; umax input double; u input double; inRange output double; tol input double; res_check_range output double
function [inRange, res_check_range] = checkInputRangeFCN(umin, umax, u, tol)

     [inRange, res_check_range] = wbc.checkInputRange(umin, umax, u, tol);
end

== matlab function MOMENTUM BASED TORQUE CONTROL/Balancing Controller QP/Compute angular momentum integral error/Select base to world transform ==
  data: state input double; booleanState output double
function booleanState = footOnGround(state)

    % output: a boolean variable whose value is 1 if the foot on ground is left
    % foot, and 0 if the foot on ground is the right foot. If both feet are on
    % ground, the variable is setted to 1.

    % states in which right foot is on ground: 9,10,11,12 (HARD CODED)
    booleanState = 1;

    if state == 9 || state == 10 || state == 11 || state == 12

        booleanState = 0;
    end
end

== matlab function MOMENTUM BASED TORQUE CONTROL/Balancing Controller QP/Compute angular momentum integral error/Get Equivalent Base Velocity ==
  data: J_l_sole input double; J_r_sole input double; feetContactStatus input double; jointPos_err input double; baseVel_equivalent output double; Reg parameter double
function baseVel_equivalent = getEquivalentBaseVel_FCN(J_l_sole, J_r_sole, feetContactStatus, jointPos_err, Reg)

    if feetContactStatus(1) == 1
    
        pinvJb             = (J_l_sole(:,1:6)'*J_l_sole(:,1:6) + Reg.pinvDamp_baseVel*eye(6))\J_l_sole(:,1:6)';
        baseVel_equivalent = -pinvJb*J_l_sole(:,7:end)*jointPos_err;
    else
        pinvJb             = (J_r_sole(:,1:6)'*J_r_sole(:,1:6) + Reg.pinvDamp_baseVel*eye(6))\J_r_sole(:,1:6)';
        baseVel_equivalent = -pinvJb*J_r_sole(:,7:end)*jointPos_err;
    end
end

== matlab function MOMENTUM BASED TORQUE CONTROL/Balancing Controller QP/Compute Desired Torques/QPSolver/QP Two Feet/Analytical Solution Two Feet (unconstrained) ==
  data: H input double; analyticalSolution output double; g input double
function analyticalSolution = analyticalSolutionQP_FCN(H,g)

    analyticalSolution = wbc.analyticalSolutionQP(H,g);
end

== matlab function MOMENTUM BASED TORQUE CONTROL/Balancing Controller QP/Compute Desired Torques/QPSolver/QP Two Feet/Process QP output ==
  data: analyticalSolution input double; primalSolution input double; QPStatus input double; f_star output double; Config parameter double
function f_star = processOutputQP_twoFeetFCN(analyticalSolution,primalSolution,QPStatus,Config)

     f_star = processOutputQP_twoFeet(analyticalSolution,primalSolution,QPStatus,Config);
end

== matlab function MOMENTUM BASED TORQUE CONTROL/Balancing Controller QP/Compute Desired Torques/QPSolver/QP One Foot/Analytical Solution QP One Foot (unconstrained) ==
  data: H input double; analyticalSolution output double; g input double
function analyticalSolution = analyticalSolutionQP_FCN(H,g)

    analyticalSolution = wbc.analyticalSolutionQP(H,g);
end

== matlab function MOMENTUM BASED TORQUE CONTROL/Balancing Controller QP/Compute Desired Torques/QPSolver/QP One Foot/Process QP output ==
  data: analyticalSolution input double; primalSolution input double; QPStatus input double; feetContactStatus input double; f_star output double; Config parameter double
function  f_star = processOutputQP_oneFoot(analyticalSolution,primalSolution,QPStatus,feetContactStatus,Config)

      f_star = processOutputQP_oneFoot(analyticalSolution,primalSolution,QPStatus,feetContactStatus,Config);
end
